simulink model "schemat1"  (R2022a)
settings: Solver=VariableStepAuto  StartTime=0.0  StopTime=100  RelTol=1e-3
values from neighbouring files (symbols this model uses):
  K = 3    [dane.m]    (also in k_stat.m = (111*ul)/50 - (171*ul.^2)/100 - (12*ul.^3)/5 + 117/100; untitled.m)
  L1 = 0.39    [dane.m]    (also in untitled.m)
  L2 = 0.37    [dane.m]    (also in untitled.m)
  L3 = -0.19    [dane.m]    (also in untitled.m)
  L4 = -0.2    [dane.m]    (also in untitled.m)
  T1 = 6    [dane.m]    (also in untitled.m)
  T2 = 7    [dane.m]    (also in untitled.m)
settings Model: Creator=danie  LastModifiedBy=danie

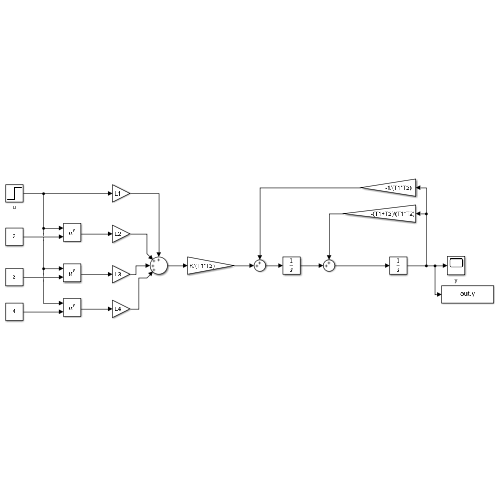
[thumbnail: Simulink's stored preview of the top-level diagram]
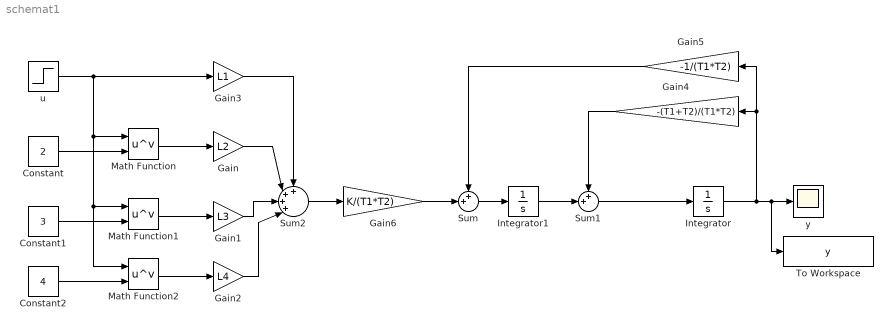
== system schemat1 ==
  Constant : Constant  Value=2
  Constant1 : Constant  Value=3
  Constant2 : Constant  Value=4
  Gain : Gain  Gain=L2
  Gain1 : Gain  Gain=L3
  Gain2 : Gain  Gain=L4
  Gain3 : Gain  Gain=L1
  Gain4 : Gain  Gain=-(T1+T2)/(T1*T2)
  Gain5 : Gain  Gain=-1/(T1*T2)
  Gain6 : Gain  Gain=K/(T1*T2)
  Integrator : Integrator
  Integrator1 : Integrator
  Math Function : Math  Operator=pow
  Math Function1 : Math  Operator=pow
  Math Function2 : Math  Operator=pow
  Sum : Sum  Inputs=++|
  Sum1 : Sum  Inputs=++|
  Sum2 : Sum  Inputs=++++|
  To Workspace : ToWorkspace  VariableName=y  SaveFormat=Structure With Time  SampleTime=-1
  u : Step  SampleTime=0
  y : Scope
  wires:
  Constant/1 -> Math Function/2
  Constant1/1 -> Math Function1/2
  Constant2/1 -> Math Function2/2
  Integrator/1 -> Gain4/1, Gain5/1, To Workspace/1, y/1
  Gain4/1 -> Sum1/1
  Sum1/1 -> Integrator/1
  Integrator1/1 -> Sum1/2
  Gain5/1 -> Sum/1
  Sum/1 -> Integrator1/1
  Gain6/1 -> Sum/2
  Math Function/1 -> Gain/1
  Math Function1/1 -> Gain1/1
  Math Function2/1 -> Gain2/1
  Sum2/1 -> Gain6/1
  Gain3/1 -> Sum2/1
  Gain/1 -> Sum2/2
  Gain1/1 -> Sum2/3
  Gain2/1 -> Sum2/4
  u/1 -> Gain3/1, Math Function2/1, Math Function1/1, Math Function/1
